simulink model "sim"  (R2025a)
settings: Solver=VariableStepAuto  StartTime=0.0  StopTime=10  RelTol=1e-3
values from neighbouring files (symbols this model uses):
  D = 0.25    [lw6.m]
  i_p = n_nom/n_rpm    (= 14.0622222222)    [lw6.m]
  J_gv = ro_gv*pi*(D/2)^4*h/2    (= 0.0118116520667)    [lw6.m]
  J_sum = 35.9e-7    (= 3.59e-06)    [lw6.m]
  k1 = 0.194    [lw6.m]
  k2 = 0.032    [lw6.m]
  k_m = 19.9e-3    (= 0.0199)    [lw6.m]
  L_a = 0.070e-3    (= 7e-05)    [lw6.m]
  R_a = 0.358    [lw6.m]
  ro = 1000    [lw6.m]
  U_nom = 18    [lw6.m]
  w_0 = n_0 * 2 * pi / 60    (= 899.542696478)    [lw6.m]
libraries: simulink x1
settings Model: Creator=user  LastModifiedBy=user

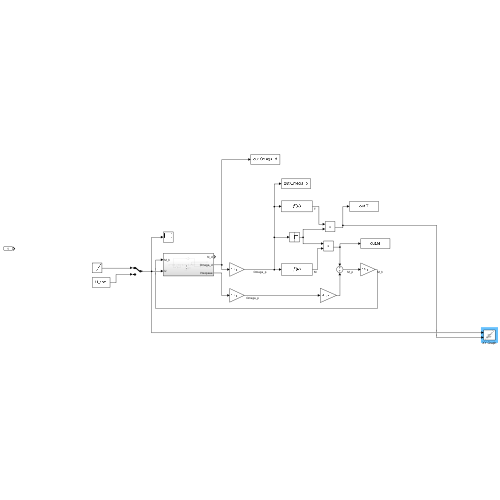
[thumbnail: Simulink's stored preview of the top-level diagram]
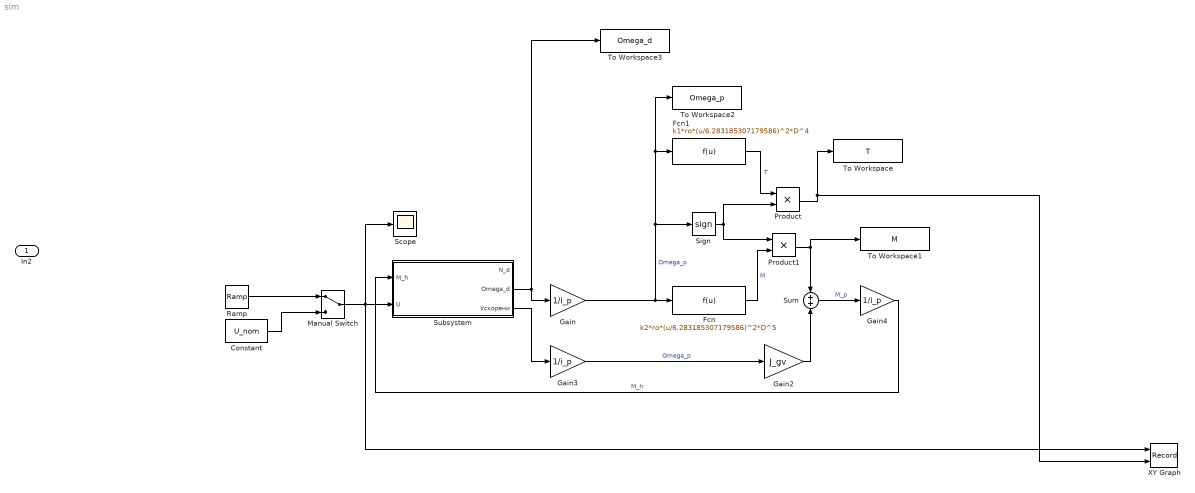
== system sim ==
  In2 : Inport
  Constant : Constant  Value=U_nom
  Fcn : Fcn  Expr=k2*ro*(u/6.283185307179586)^2*D^5
  Fcn1 : Fcn  Expr=k1*ro*(u/6.283185307179586)^2*D^4
  Gain : Gain  Gain=1/i_p
  Gain2 : Gain  Gain=J_gv
  Gain3 : Gain  Gain=1/i_p
  Gain4 : Gain  Gain=1/i_p
  Manual Switch : ManualSwitch
  Product : Product
  Product1 : Product
  Ramp : simulink/Sources/Ramp  slope=36/10  start=0  InitialOutput=-18
  Scope : Scope
      settings: ActiveDisplayYMinimum=-1  ActiveDisplayYMaximum=1
  Sign : Signum
  Subsystem : Subsystem
  Sum : Sum
  To Workspace : ToWorkspace  VariableName=T  SaveFormat=Timeseries  SampleTime=-1
  To Workspace1 : ToWorkspace  VariableName=M  SaveFormat=Timeseries  SampleTime=-1
  To Workspace2 : ToWorkspace  VariableName=Omega_p  SaveFormat=Timeseries  SampleTime=-1
  To Workspace3 : ToWorkspace  VariableName=Omega_d  SaveFormat=Timeseries  SampleTime=-1
  XY Graph : Record  NumPorts=2.0  FileSettingsInternal="{\"entries\":[{\"content\":{\"excelSettings\":{\"content\":{},\"type\":\"Streamout.ExcelSettings\"},\"parquetSettings\":{\"content\":{},\"type\":\"Streamout.ParquetSettings\"}},\"type\":\"Streamout.FileSettingStorage\",\"uuid\":\"\"}],\"packageUris\":[\"http:\\/\\/schema.mathworks.com\\/mf0\\/streamout_blocks\\/R2020a\"],\"version\":\"1.0\"}"  FrameSettings=[0, 0]  Layout=[1 1]  SignalsInternal="{\"entries\":[{\"content\":{\"signals\":[{\"content\":{\"blockPath\":[],\"dimensions\":[1],\"domain\":\"\",\"lineColor\":\"#a2142f\",\"plots\":[ 1 ],\"port\":1,\"sid\":[\"\"],\"signalID\":1,\"signalName\":\"Manual Switch\"},\"type\":\"RecordBlkView.Signal\",\"uuid\":\"\"},{\"content\":{\"blockPath\":[],\"dimensions\":[1],\"domain\":\"\",\"lineColor\":\"#139fff\",\"plots\":[ 1 ],\"port\":2,\"sid\":[\"\"],\"signalID\":2,\"signalName\":\"Product\"},\"type\":\"RecordBlkView.Signal\",\"uuid\":\"\"}]},\"type\":\"RecordBlkView.InputSignals\",\"uuid\":\"\"}],\"packageUris\":[\"http:\\/\\/schema.mathworks.com\\/mf0\\/streamout_blocks\\/R2020a\"],\"version\":\"1.0\"}"  VisualizationBindings="{\"xyplotplugin\":{\"info\":[{\"series\":[{\"bindingParametersList\":[{\"parameter\":\"X-Axis\",\"signalID\":1,\"signalName\":\"Manual Switch\"},{\"parameter\":\"Y-Axis\",\"signalID\":2,\"signalName\":\"Product\"}],\"seriesID\":0}],\"subplotID\":1}]}}"  CompatibilityTag=XY
  wires:
  Ramp/1 -> Manual Switch/1
  Constant/1 -> Manual Switch/2
  Manual Switch/1 -> Scope/1, XY Graph/1, Subsystem/2(U)
  Subsystem/2(Omega_d) -> Gain/1, To Workspace3/1
  Gain/1 -> Fcn/1, To Workspace2/1, Fcn1/1, Sign/1  "Omega_p"
  Fcn/1 -> Product1/2  "M"
  Gain2/1 -> Sum/2
  Sum/1 -> Gain4/1  "M_p"
  Fcn1/1 -> Product/1  "T"
  Gain3/1 -> Gain2/1  "Omega_p"
  Subsystem/3(Ускорени) -> Gain3/1
  Gain4/1 -> Subsystem/1(M_h)  "M_h"
  Sign/1 -> Product/2, Product1/1
  Product1/1 -> Sum/1, To Workspace1/1
  Product/1 -> To Workspace/1, XY Graph/2

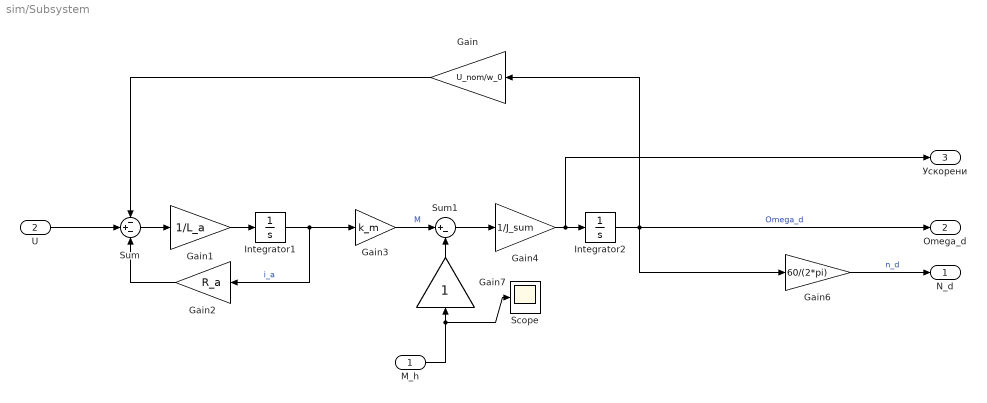
== system sim/Subsystem ==
  M_h : Inport
  U : Inport  Port=2
  Gain : Gain  Gain=U_nom/w_0
  Gain1 : Gain  Gain=1/L_a
  Gain2 : Gain  Gain=R_a
  Gain3 : Gain  Gain=k_m
  Gain4 : Gain  Gain=1/J_sum
  Gain6 : Gain  Gain=60/(2*pi)
  Gain7 : Gain
  Integrator1 : Integrator
  Integrator2 : Integrator
  Scope : Scope
      settings: ActiveDisplayYMinimum=-1  ActiveDisplayYMaximum=1
  Sum : Sum  Inputs=-+-
  Sum1 : Sum  Inputs=|+-
  N_d : Outport
  Omega_d : Outport  Port=2
  Ускорени : Outport  Port=3
  wires:
  U/1 -> Sum/2
  Gain3/1 -> Sum1/1  "M"
  M_h/1 -> Scope/1, Gain7/1
  Gain6/1 -> N_d/1  "n_d"
  Gain1/1 -> Integrator1/1
  Integrator1/1 -> Gain3/1, Gain2/1  "i_a"
  Integrator2/1 -> Omega_d/1, Gain6/1, Gain/1  "Omega_d"
  Gain4/1 -> Ускорени/1, Integrator2/1
  Sum/1 -> Gain1/1
  Gain2/1 -> Sum/3
  Gain7/1 -> Sum1/2
  Gain/1 -> Sum/1
  Sum1/1 -> Gain4/1
